simulink subsystem "ADC_Model_SILPIL_atomic"  (R2022a)
settings: Solver=VariableStepAuto  StartTime=0.0  StopTime=10.0  RelTol=1e-3
model mask{Out_Mode=0, Gain=0, Offset=0, Vcc=0, ADCBit=12, PGA_Gain=1}
  mask prompts: Out_Mode "Output Mode"
settings Model: Creator=BEDNASA  LastModifiedBy=BEDNASA

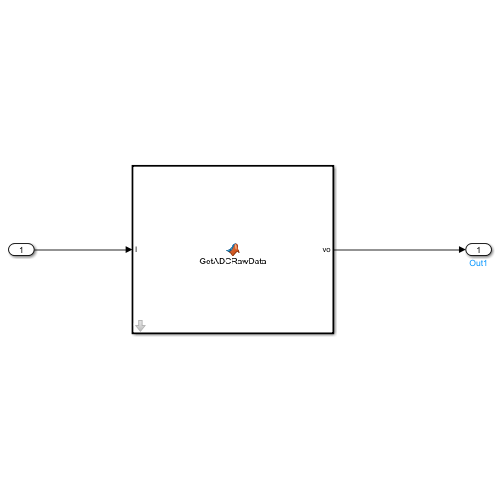
[thumbnail: Simulink's stored preview of the top-level diagram]
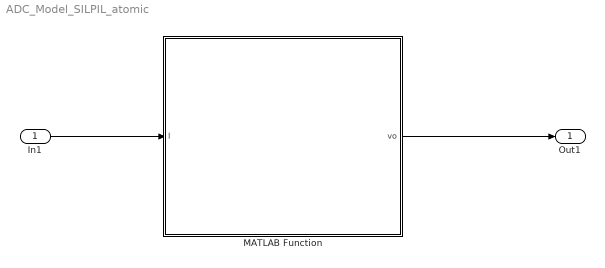
== system ADC_Model_SILPIL_atomic ==
  In1 : Inport
  MATLAB Function : MATLAB Function  TreatAsAtomicUnit=on  mask(ADC model){Out_Mode=Out_Mode, Gain=Gain, Offset=Offset, Vcc=Vcc, ADCBit=ADCBit, PGA_Gain=PGA_Gain}
      mask prompts: Out_Mode "Output Mode"
      mask help: Atomic ADC model utlized in custom blocks for single and three phase drive systems
  Out1 : Outport
  wires:
  In1/1 -> MATLAB Function/1(I)
  MATLAB Function/1(vo) -> Out1/1

== matlab function ADC_Model_SILPIL_atomic/MATLAB Function ==
  data: I input; vo output; Gain parameter; Offset parameter; Vcc parameter; ADCBit parameter; PGA_Gain parameter; Out_Mode parameter
function vo = GetADCRawData(I, Gain, Offset, Vcc, ADCBit, PGA_Gain, Out_Mode)

%Vcc = 1;
%out_mode = 0;
%ADCBit = 12;


%Vout = C1*I+C2;
%Vout_PIL = 1;

Vout=Gain * I + Offset;
Vout_PIL = (Gain/PGA_Gain) * I + Offset/PGA_Gain;

if (Vout > Vcc)
    Vout = Vcc;
elseif (Vout < 0)
    Vout = 0;
end

if Out_Mode == 0        % ADC_counts
    vo = round((Vout/Vcc) * (2^ADCBit));
elseif Out_Mode == 1    % ADC_voltage
    vo = Vout_PIL;
else 
    vo = 0;
end


% function AD_count  = GetADCRawData(in_analog, Gain, Offset, Vcc, ADCbit)
% %% Sensor model with ADC
% % Sensor voltage equation V_out = Gain * in_analog + Offset
% 
% V_out = Gain * in_analog + Offset;
% 
% if (V_out > Vcc)
%     V_out = Vcc;
% elseif (V_out < 0)
%     V_out = 0;
% end
% 
% %% AD Counts
% AD_count = round((V_out/Vcc) * (2^ADCbit));
% end
